simulink model "dynamics_aquad"  (R2016a)
settings: Solver=VariableStepAuto  StartTime=0.0  StopTime=10  RelTol=1e-3
model workspace (MAT data in the model file):
  B = Simulink.Signal
  B.DataType = 'double'
  B.Dimensions = 1
  B.DimensionsMode = 'auto'
  B.Complexity = 'real'
  B.SampleTime = -1
  B.SamplingMode = 'auto'
  W = Simulink.Signal
  W.DataType = 'double'
  W.Dimensions = 1
  W.DimensionsMode = 'auto'
  W.Complexity = 'real'
  W.SampleTime = -1
  W.SamplingMode = 'auto'
  rho = Simulink.Signal
  rho.DataType = 'double'
  rho.Dimensions = 1
  rho.DimensionsMode = 'auto'
  rho.Complexity = 'real'
  rho.SampleTime = -1
  rho.SamplingMode = 'auto'
  xb = Simulink.Signal
  xb.DataType = 'double'
  xb.Dimensions = 1
  xb.DimensionsMode = 'auto'
  xb.Complexity = 'real'
  xb.SampleTime = -1
  xb.SamplingMode = 'auto'
  xg = Simulink.Signal
  xg.DataType = 'double'
  xg.Dimensions = 1
  xg.DimensionsMode = 'auto'
  xg.Complexity = 'real'
  xg.SampleTime = -1
  xg.SamplingMode = 'auto'
  yb = Simulink.Signal
  yb.DataType = 'double'
  yb.Dimensions = 1
  yb.DimensionsMode = 'auto'
  yb.Complexity = 'real'
  yb.SampleTime = -1
  yb.SamplingMode = 'auto'
  yg = Simulink.Signal
  yg.DataType = 'double'
  yg.Dimensions = 1
  yg.DimensionsMode = 'auto'
  yg.Complexity = 'real'
  yg.SampleTime = -1
  yg.SamplingMode = 'auto'
  zb = Simulink.Signal
  zb.DataType = 'double'
  zb.Dimensions = 1
  zb.DimensionsMode = 'auto'
  zb.Complexity = 'real'
  zb.SampleTime = -1
  zb.SamplingMode = 'auto'
  zg = Simulink.Signal
  zg.DataType = 'double'
  zg.Dimensions = 1
  zg.DimensionsMode = 'auto'
  zg.Complexity = 'real'
  zg.SampleTime = -1
  zg.SamplingMode = 'auto'
values from neighbouring files (symbols this model uses):
  Thrust_vs_PWM = [-40.03398 -39.589158 -38.699514 -37.5429768 -36.6088506 -35.4967956 -33.7619898 -32.3830416 -31.2265044 -29.9810028 -28.5130902 -27.6234462 ... (243 elements, 81x3)]    [Thrust_PWM.mat]
undefined symbols (not defined in the file or in its folder): alpha_AoA
settings Model: Creator=ridhi  LastModifiedBy=lenovo

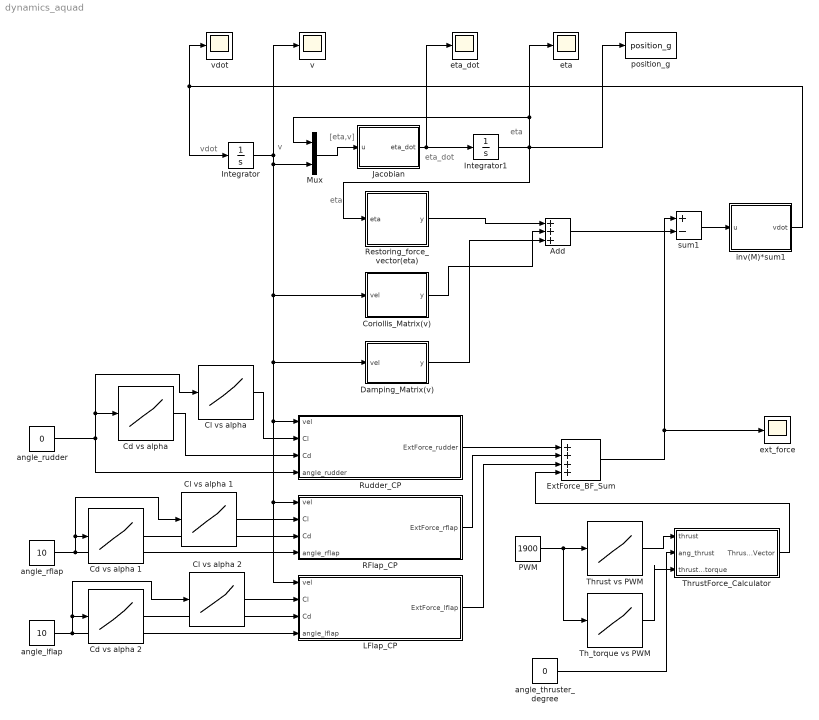
== system dynamics_aquad ==
  note: vdot
  note: eta
  note: v
  note: eta
  note: eta_dot
  note: [eta,v]
  Add : Sum  Inputs=+++
  "Cd vs alpha " : Lookup_n-D  NumberOfTableDimensions=1  BreakpointsForDimension1=alpha_AoA(:,1)  Table=alpha_AoA(:,2)  InternalRulePriority=Speed  RndMeth=Simplest  InputSameDT=on
  Cd vs alpha 1 : Lookup_n-D  NumberOfTableDimensions=1  BreakpointsForDimension1=alpha_AoA(:,1)  Table=alpha_AoA(:,2)  InternalRulePriority=Speed  RndMeth=Simplest  InputSameDT=on
  Cd vs alpha 2 : Lookup_n-D  NumberOfTableDimensions=1  BreakpointsForDimension1=alpha_AoA(:,1)  Table=alpha_AoA(:,2)  InternalRulePriority=Speed  RndMeth=Simplest  InputSameDT=on
  "Cl vs alpha " : Lookup_n-D  NumberOfTableDimensions=1  BreakpointsForDimension1=alpha_AoA(:,1)  Table=alpha_AoA(:,3)  InternalRulePriority=Speed  RndMeth=Simplest  InputSameDT=on
  Cl vs alpha 1 : Lookup_n-D  NumberOfTableDimensions=1  BreakpointsForDimension1=alpha_AoA(:,1)  Table=alpha_AoA(:,3)  InternalRulePriority=Speed  RndMeth=Simplest  InputSameDT=on
  Cl vs alpha 2 : Lookup_n-D  NumberOfTableDimensions=1  BreakpointsForDimension1=alpha_AoA(:,1)  Table=alpha_AoA(:,3)  InternalRulePriority=Speed  RndMeth=Simplest  InputSameDT=on
  Coriollis_Matrix(v) : MATLAB Function  TreatAsAtomicUnit=on
  Damping_Matrix(v) : MATLAB Function  TreatAsAtomicUnit=on
  ExtForce_BF_Sum : Sum  Inputs=++++
  Integrator : Integrator  InitialCondition=[0;0;0;0;0;0]
  Integrator1 : Integrator  InitialCondition=[0;0;0;0;0;0]  LimitOutput=on
  Jacobian : MATLAB Function  TreatAsAtomicUnit=on
  LFlap_CP : MATLAB Function  TreatAsAtomicUnit=on
  Mux : Mux  Inputs=2
  PWM : Constant  Value=1900
  RFlap_CP : MATLAB Function  TreatAsAtomicUnit=on
  Restoring_force_vector(eta) : MATLAB Function  TreatAsAtomicUnit=on
  Rudder_CP : MATLAB Function  TreatAsAtomicUnit=on
  Th_torque vs PWM : Lookup_n-D  NumberOfTableDimensions=1  BreakpointsForDimension1=Thrust_vs_PWM(:,2)  BreakpointsForDimension2=Thrust_vs_PWM(:,3)  Table=Thrust_vs_PWM(:,3)  InternalRulePriority=Speed  RndMeth=Simplest  InputSameDT=on
  Thrust vs PWM : Lookup_n-D  NumberOfTableDimensions=1  BreakpointsForDimension1=Thrust_vs_PWM(:,2)  BreakpointsForDimension2=Thrust_vs_PWM(:,3)  Table=Thrust_vs_PWM(:,1)  InternalRulePriority=Speed  RndMeth=Simplest  InputSameDT=on
  ThrustForce_Calculator : MATLAB Function  TreatAsAtomicUnit=on
  angle_lflap : Constant  Value=10
  angle_rflap : Constant  Value=10
  angle_rudder : Constant  Value=0
  angle_thruster_degree : Constant  Value=0
  eta : Scope
  eta_dot : Scope
  ext_force : Scope
  inv(M)*sum1 : MATLAB Function  TreatAsAtomicUnit=on
  position_g : ToWorkspace  VariableName=position_g  SaveFormat=Timeseries  SampleTime=-1
  sum1 : Sum  Inputs=+-
  "v " : Scope
  vdot : Scope
  wires:
  Mux/1 -> Jacobian/1(u)
  Jacobian/1(eta_dot) -> eta_dot/1, Integrator1/1
  Restoring_force_vector(eta)/1(y) -> Add/1
  Coriollis_Matrix(v)/1(y) -> Add/2
  Damping_Matrix(v)/1(y) -> Add/3
  Add/1 -> sum1/2
  inv(M)*sum1/1(vdot) -> Integrator/1, vdot/1
  sum1/1 -> inv(M)*sum1/1(u)
  Integrator/1 -> Mux/2, LFlap_CP/1(vel), RFlap_CP/1(vel), Rudder_CP/1(vel), Damping_Matrix(v)/1(vel), Coriollis_Matrix(v)/1(vel), "v "/1
  angle_rudder/1 -> "Cl vs alpha "/1, "Cd vs alpha "/1, Rudder_CP/4(angle_rudder)
  angle_rflap/1 -> Cl vs alpha 1/1, Cd vs alpha 1/1, RFlap_CP/4(angle_rflap)
  "Cd vs alpha "/1 -> Rudder_CP/3(Cd)
  "Cl vs alpha "/1 -> Rudder_CP/2(Cl)
  Rudder_CP/1(ExtForce_rudder) -> ExtForce_BF_Sum/1
  RFlap_CP/1(ExtForce_rflap) -> ExtForce_BF_Sum/2
  LFlap_CP/1(ExtForce_lflap) -> ExtForce_BF_Sum/3
  ExtForce_BF_Sum/1 -> sum1/1, ext_force/1
  Integrator1/1 -> eta/1, Mux/1, position_g/1, Restoring_force_vector(eta)/1(eta)
  Cd vs alpha 1/1 -> RFlap_CP/3(Cd)
  Cl vs alpha 1/1 -> RFlap_CP/2(Cl)
  Cd vs alpha 2/1 -> LFlap_CP/3(Cd)
  Cl vs alpha 2/1 -> LFlap_CP/2(Cl)
  angle_lflap/1 -> Cl vs alpha 2/1, Cd vs alpha 2/1, LFlap_CP/4(angle_lflap)
  PWM/1 -> Th_torque vs PWM/1, Thrust vs PWM/1
  ThrustForce_Calculator/1(ThrusterForceVector) -> ExtForce_BF_Sum/4
  Thrust vs PWM/1 -> ThrustForce_Calculator/1(thrust)
  angle_thruster_degree/1 -> ThrustForce_Calculator/2(ang_thrust)
  Th_torque vs PWM/1 -> ThrustForce_Calculator/3(thruster_torque)

== matlab function dynamics_aquad/Coriollis_Matrix(v) ==
  data: vel input; y output; xg data_store_memory; yg data_store_memory; zg data_store_memory; W data_store_memory
function y = fcn(vel)
u = vel(1);
v = vel(2);
w = vel(3);
p = vel(4);
q = vel(5);
r = vel(6);
global xg yg zg W
m=W/9.81;
Ix = 141; Iy = 3895; Iz = 4036; Ixy = 0; Ixz = 0; Iyx = 0; Izy = 0; Izx = 0; Iyz = 0; 

Xudot = -321.3; Xvdot =0; Xwdot=0; Xpdot=0; Xqdot=0; Xrdot=0;
Yudot = -1049.2; Yvdot =0; Ywdot=0; Ypdot=0; Yqdot=0; Yrdot=-996.04;
Zudot = 0; Zvdot =0; Zwdot=-7040.4; Zpdot=0; Zqdot=-277.2; Zrdot=0;
Kudot = 0; Kvdot =0; Kwdot=0; Kpdot=0; Kqdot=0; Krdot=0;
Mudot = 0; Mvdot =0; Mwdot=0; Mpdot=0; Mqdot=-7045.3; Mrdot=0;
Nudot = 0; Nvdot =0; Nwdot=0; Npdot=0; Nqdot=0; Nrdot=-8584.2;

a1 = [Xudot Xvdot Xwdot Xpdot Xqdot Xrdot]*vel;
a2 = [Yudot Yvdot Ywdot Ypdot Yqdot Yrdot]*vel;
a3 = [Zudot Zvdot Zwdot Zpdot Zqdot Zrdot]*vel;
b1 = [Kudot Kvdot Kwdot Kpdot Kqdot Krdot]*vel;
b2 = [Mudot Mvdot Mwdot Mpdot Mqdot Mrdot]*vel;
b3 = [Nudot Nvdot Nwdot Npdot Nqdot Nrdot]*vel;


C_rb=[ 0                0              0              m *(yg*q+zg*r)        -m*(xg*q-w)             -m*(xg*r+v);
       0                0              0             -m*(yg*p+w)             m*(zg*r+xg*p)          -m*(yg*r-u);
       0                0              0             -m*(zg*p-v)            -m*(zg*q+u)             m*(xg*p+yg*q);
       -m *(yg*q+zg*r)  m*(yg*p+w)     m*(zg*p-v)     0                      -Iyz*q-Ixz*p+Iz*r       Iyz*r+Ixy*p-Iy*q;
       m*(xg*q-w)      -m*(zg*r+xg*p)  m*(zg*q+u)     Iyz*q+Ixz*p-Iz*r             0                  -Ixz*r-Ixy*q+Ix*p;
       m*(xg*r+v)       m*(yg*r-u)    -m*(xg*p+yg*q) -Iyz*r-Ixy*p+Iy*q       Ixz*r+Ixy*q-Ix*p               0            ];
 
C_a= [0    0    0   0   -a3    a2
      0    0    0   a3    0   -a1
      0    0    0   -a2   a1   0 
      0   -a3    a2  0   -b3  b2
      a3    0   -a1  b3   0   -b1
     -a2   a1   0    -b2  b1   0];

C = C_rb+C_a;
y = C*vel;
end

== matlab function dynamics_aquad/Jacobian ==
  data: u input; eta_dot output
function eta_dot = fcn(u)

v = u(7:12); %body_frame_velocities

phi=u(4); %roll
theta=u(5); %pitch
si=u(6);   %yaw
c_p=cos(phi);
c_t=cos(theta);
c_s=cos(si);
s_p=sin(phi);
s_t=sin(theta);
s_s=sin(si);
t_t=tan(theta);


J1=[c_s*c_t    -s_s*c_p+s_p*s_t*c_s     s_s*s_p+s_t*c_s*c_p;
    s_s*c_t     c_s*c_p+s_p*s_t*s_s    -c_s*s_p+s_t*s_s*c_p;
     -s_t            s_p*c_t                 c_p*c_t       ];
       
J2=[1      s_p*t_t     c_p*t_t;
    0        c_p        -s_p;
    0      s_p/c_t     c_p/c_t ];


J=[J1 zeros(3,3); zeros(3,3) J2];
eta_dot = J * v; % y == earth_velocities

end

== matlab function dynamics_aquad/Damping_Matrix(v) ==
  data: vel input; y output
function y = fcn(vel)
u = vel(1);
v = vel(2);
w = vel(3);
p = vel(4);
q = vel(5);
r = vel(6);

U = sqrt(u^2+v^2+w^2);

Xu = 37.3; Xv = -17.2; Xw=28.3; Xp=0; Xq=0; Xr=0;
Yu = 0; Yv =875.3; Yw=0; Yp=0; Yq=0; Yr=-1381.5;
Zu = 0; Zv =0; Zw=1447.3; Zp=0; Zq=2052.9; Zr=0;
Ku = 0; Kv =0; Kw=0; Kp=0; Kq=0; Kr=0;
Mu = 0; Mv =0; Mw=-3105.3; Mp=0; Mq=-6497.6; Mr=0;
Nu = 0; Nv =372.1; Nw=0; Np=0; Nq=0; Nr=1194.3;

Xuu = 13.6; Xvv = -22.6; Xww=282; Xpp=0; Xqq=0; Xrr=0;
Yuu = 0; Yvv =227.5; Yww=0; Ypp=0; Yqq=0; Yrr=0;
Zuu = 0; Zvv =0; Zww=2859.5; Zpp=0; Zqq=0; Zrr=0;
Kuu = 0; Kvv =0; Kww=0; Kpp=0; Kqq=0; Krr=0;
Muu = 0; Mvv =0; Mww=381; Mpp=0; Mqq=-7045.3; Mrr=0;
Nuu = 0; Nvv =-1006.5; Nww=0; Npp=0; Nqq=0; Nrr=0;


D_L =  U*[Xu  Xv  Xw  Xp  Xq  Xr 
          Yu  Yv  Yw  Yp  Yq  Yr 
          Zu  Zv  Zw  Zp  Zq  Zr 
          Ku  Kv  Kw  Kp  Kq  Kr 
          Mu  Mv  Mw  Mp  Mq  Mr 
          Nu  Nv  Nw  Np  Nq  Nr ];
D_Q =  U*[Xuu*abs(u) Xvv*abs(v) Xww*abs(w) Xpp*abs(p) Xqq*abs(q) Xrr*abs(r)
          Yuu*abs(u) Yvv*abs(v) Yww*abs(w) Ypp*abs(p) Yqq*abs(q) Yrr*abs(r)
          Zuu*abs(u) Zvv*abs(v) Zww*abs(w) Zpp*abs(p) Zqq*abs(q) Zrr*abs(r)
          Kuu*abs(u) Kvv*abs(v) Kww*abs(w) Kpp*abs(p) Kqq*abs(q) Krr*abs(r)
          Muu*abs(u) Mvv*abs(v) Mww*abs(w) Mpp*abs(p) Mqq*abs(q) Mrr*abs(r)
          Nuu*abs(u) Nvv*abs(v) Nww*abs(w) Npp*abs(p) Nqq*abs(q) Nrr*abs(r)];
D = D_L + D_Q;
  
y = D*vel;
end

== matlab function dynamics_aquad/Restoring_force_vector(eta) ==
  data: eta input; y output; xg data_store_memory; yg data_store_memory; zg data_store_memory; xb data_store_memory; yb data_store_memory; zb data_store_memory; W data_store_memory; B data_store_memory
function y = fcn(eta)

theta = eta(5);
phi = eta(4);
global xg yg zg W B xb yb zb

W = 6*9.91; B = 7*9.81;
xg =0; yg =0; zg =0; xb = 0; yb= 0.05;zb = 0.05;
G=   [(W-B)*sin(theta);
       -(W-B)*cos(theta)*sin(phi);
       -(W-B)*cos(theta)*cos(phi);
       -(yg*W-yb*B)*cos(theta)*cos(phi)+(zg*W-zb*B)*cos(theta)*sin(phi);
       (zg*W-zb*B)*sin(theta)+(xg*W-xb*B)*cos(theta)*cos(phi);
       -(xg*W-xb*B)*cos(theta)*sin(phi)-(yg*W-yb*B)*sin(theta)];
y =  G;

end

== matlab function dynamics_aquad/inv(M)*sum1 ==
  data: u input; vdot output; zg data_store_memory; xg data_store_memory; yg data_store_memory; W data_store_memory
function vdot = fcn(u)
sum1 = u;

global W xg yg zg
m = W/9.81;
Ix = 141; Iy = 3895; Iz = 4036; Ixy = 0; Ixz = 0; Iyx = 0; Izy = 0; Izx = 0; Iyz = 0; 
Xudot = -321.3; Xvdot =0; Xwdot=0; Xpdot=0; Xqdot=0; Xrdot=0;
Yudot = -1049.2; Yvdot =0; Ywdot=0; Ypdot=0; Yqdot=0; Yrdot=-996.04;
Zudot = 0; Zvdot =0; Zwdot=-7040.4; Zpdot=0; Zqdot=-277.2; Zrdot=0;
Kudot = 0; Kvdot =0; Kwdot=0; Kpdot=0; Kqdot=0; Krdot=0;
Mudot = 0; Mvdot =0; Mwdot=0; Mpdot=0; Mqdot=-7045.3; Mrdot=0;
Nudot = 0; Nvdot =0; Nwdot=0; Npdot=0; Nqdot=0; Nrdot=-8584.2;

M_rb=[m     0      0     0         m*zg        -m*yg;
      0     m      0    -m*zg       0        m*xg;
      0     0      m     m*yg       -m*xg       0;
      0    -m*zg m*yg     Ix        -Ixy      -Ixz;
     m*zg    0   -m*xg  -Iyx        Iy      -Iyz;
    -m*yg  m*xg   0    -Izx       -Izy      Iz];
  
M_a=-[Xudot Xvdot Xwdot Xpdot Xqdot Xrdot
      Yudot Yvdot Ywdot Ypdot Yqdot Yrdot
      Zudot Zvdot Zwdot Zpdot Zqdot Zrdot
      Kudot Kvdot Kwdot Kpdot Kqdot Krdot
      Mudot Mvdot Mwdot Mpdot Mqdot Mrdot
      Nudot Nvdot Nwdot Npdot Nqdot Nrdot];
 
M=M_rb+M_a; 

vdot = inv(M)*sum1;

end

== matlab function dynamics_aquad/Rudder_CP ==
  data: vel input; ExtForce_rudder output; Cl input; Cd input; rho data_store_memory; angle_rudder input
function ExtForce_rudder = fcn(vel,Cl,Cd,angle_rudder)

u = vel(1);
global rho
rho = 1000;
A_rudder = 0.02;
a = 100; b= 200; rx = 135; rz =60; ry = 0;
angle_rad = angle_rudder*(pi/180);

D = (1/2)*Cl*rho*A_rudder*u^2;
L = (1/2)*Cd*rho*A_rudder*u^2;
Fx = -(D*cos(angle_rad)+L*sin(angle_rad));
Fy =  (D*sin(angle_rad)-L*cos(angle_rad));
Fz =  0;
Mx = -Fy*(rz+(a/2));
My =  Fx*(rz+(a/2));
Mz =  Fx*(b/2)*sin(angle_rad)+Fy*(rx+(a/2));

ExtForce_rudder = [Fx;Fy;Fz;Mx;My;Mz];

end

== matlab function dynamics_aquad/RFlap_CP ==
  data: vel input; ExtForce_rflap output; Cl input; Cd input; rho data_store_memory; angle_rflap input
function ExtForce_rflap = fcn(vel,Cl,Cd,angle_rflap)

u = vel(1);
global rho
rho = 1000;

A_rflap = 0.015;
a = 100; b= 150; rx = 90; rz = 30; ry = 88;
angle_rad = angle_rflap*(pi/180);

D = (1/2)*Cl*rho*A_rflap*u^2;
L = (1/2)*Cd*rho*A_rflap*u^2;
Fx = -(D*cos(angle_rad)+L*sin(angle_rad));
Fy =  0;
Fz =  (D*sin(angle_rad)-L*cos(angle_rad));
Mx =  Fz*(ry+(a/2));
My =  Fx*(rz+(b/2)*sin(angle_rad))+Fz*(rx+(b/2)*cos(angle_rad));
Mz =  Fx*(ry+(a/2));

ExtForce_rflap = [Fx;Fy;Fz;Mx;My;Mz];

end

== matlab function dynamics_aquad/LFlap_CP ==
  data: vel input; ExtForce_lflap output; Cl input; Cd input; rho data_store_memory; angle_lflap input
function ExtForce_lflap = fcn(vel,Cl,Cd,angle_lflap)

u = vel(1);
global rho
rho = 1000;

A_lflap = 0.015;
a = 100; b= 150; rx = 90; rz = 30; ry = 88;
angle_rad = angle_lflap*(pi/180);

D = (1/2)*Cl*rho*A_lflap*u^2;
L = (1/2)*Cd*rho*A_lflap*u^2;
Fx = -(D*cos(angle_rad)+L*sin(angle_rad));
Fy =  0;
Fz =  (D*sin(angle_rad)-L*cos(angle_rad));
Mx = -(Fz*(ry+(a/2)));
My =  Fx*(rz+(b/2)*sin(angle_rad))+Fz*(rx+(b/2)*cos(angle_rad));
Mz = -(Fx*(ry+(a/2)));

ExtForce_lflap = [Fx;Fy;Fz;Mx;My;Mz];

end

== matlab function dynamics_aquad/ThrustForce_Calculator ==
  data: thrust input; ThrusterForceVector output; ang_thrust input; thruster_torque input
function ThrusterForceVector = fcn(thrust,ang_thrust,thruster_torque)

ang_rad_th = ang_thrust*(pi/180);
zth=0.07;
xth=0.02;
Mth=thruster_torque;

Fx = thrust*cos(ang_rad_th);
Fy = 0;
Fz = thrust*sin(ang_rad_th);
Mx = Mth*cos(ang_rad_th);
My = Fx*zth+Fz*xth;
Mz = Mth*sin(ang_rad_th); 


ThrusterForceVector = [Fx;Fy;Fz;Mx;My;Mz];

end
